simulink model "TestFrottementsNew"  (Simulink 6.5)
settings: Solver=ode45  StartTime=0.0  StopTime=TimeTqStop  MaxStep=0.1  RelTol=1e-3
undefined symbols (not defined in the file): RegimeTq, TempsTq, TorqueLosesTest, TorqueLosesTimeTest, x
settings Model: Creator=a030141  LastModifiedBy=Zeus
settings DataIOCC: SignalLoggingName=sigsOut
settings DebuggingCC: SolverPrmCheckMsg=none  MultiTaskDSMMsg=warning  MultiTaskCondExecSysMsg=none  StrictBusMsg=None
settings HardwareCC: TargetUnknown=on
settings RTWCC: IncludeERTFirstTime=on

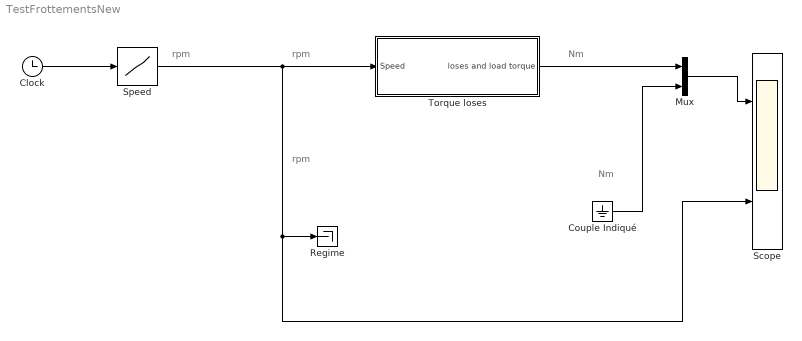
== system TestFrottementsNew ==
  note: Nm
  note: rpm
  note: rpm
  note: rpm
  note: Nm
  " Torque loses" : Subsystem
  Clock : Clock
      settings: Decimation=10
  Couple Indiqué : Ground
  Mux : Mux  Inputs=2
  Regime : Terminator
  Scope : Scope  NumInputPorts=2
      settings: YMin=-5~-5  YMax=5~5
  Speed : Lookup  InputValues=TempsTq  OutputValues=RegimeTq  LookUpMeth=Interpolation-Extrapolation  OutDataType=sfix(16)  OutScaling=2^0  SaturateOnIntegerOverflow=on  SampleTime=-1  LUTDesignTableMode=Redesign Table  LUTDesignDataSource=Block Dialog  LUTDesignFunctionName=sqrt(x)  LUTDesignUseExistingBP=on  LUTDesignRelError=0.01  LUTDesignAbsError=1e-6  RndMeth=Floor
      settings: LockScale=off
  wires:
  Clock/1 -> Speed/1
  Speed/1 -> Regime/1, Scope/2, " Torque loses"/1(Speed)
  Mux/1 -> Scope/1
  " Torque loses"/1(loses and load torque) -> Mux/1
  Couple Indiqué/1 -> Mux/2

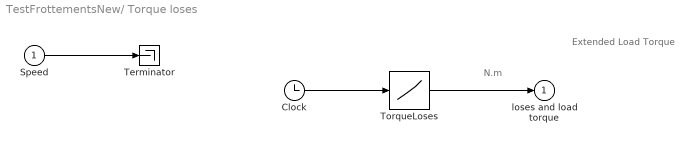
== system TestFrottementsNew/ Torque loses ==
  note: N.m
  note: Extended Load Torque
  Speed : Inport
  Clock : Clock
      settings: Decimation=10
  Terminator : Terminator
  TorqueLoses : Lookup  InputValues=TorqueLosesTimeTest  OutputValues=TorqueLosesTest  LookUpMeth=Interpolation-Extrapolation  OutDataType=sfix(16)  OutScaling=2^0  SaturateOnIntegerOverflow=on  SampleTime=-1  LUTDesignTableMode=Redesign Table  LUTDesignDataSource=Block Dialog  LUTDesignFunctionName=sqrt(x)  LUTDesignUseExistingBP=on  LUTDesignRelError=0.01  LUTDesignAbsError=1e-6  RndMeth=Floor
      settings: LockScale=off
  loses and load torque : Outport
  wires:
  Clock/1 -> TorqueLoses/1
  TorqueLoses/1 -> loses and load torque/1
  Speed/1 -> Terminator/1
